simulink model "RI_RL_PI_MRZK_DI"  (R2013b)
settings: Solver=ode45  StartTime=0.0  StopTime=25*L/R  MaxStep=tau/100  RelTol=1e-3
InitFcn:
  | % Modellparaméterek
  | R = 250e-3;
  | L = 10e-3;
  | Psi_0 = 0.5e-3;
  | 
  | i_0 = 0;
  | theta_0 = 0;
  | 
  | % Rendszerparaméterek
  | K = 1/R;
  | tau = L/R;
  | 
  | % PI-hangolás
  | tau_CL = tau/25;
  | xi_CL = 1;
  | 
  | K_PI = (2*xi_CL*tau - tau_CL)/(K*tau_CL);
  | T_I = (2*xi_CL*tau - tau_CL)*tau_CL/tau;
libraries: RI_MK x5, simulink x1
settings Model: Creator=Szalay  LastModifiedBy=Szalay

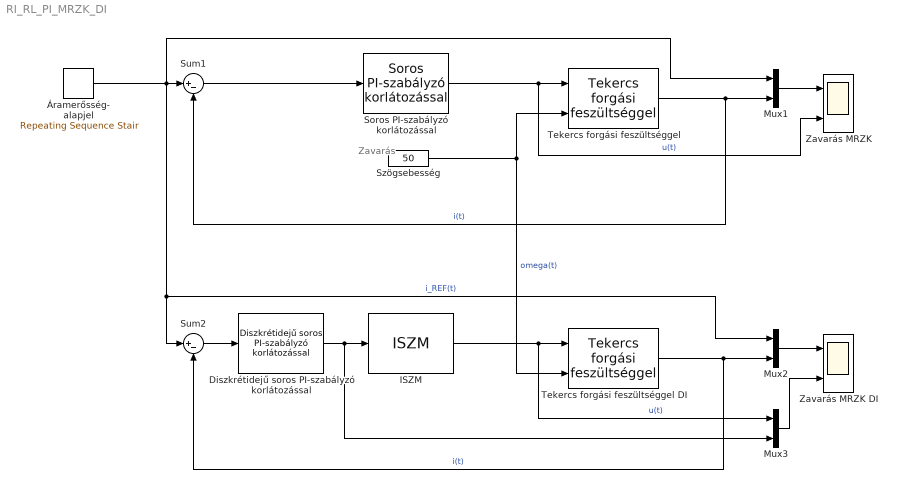
== system RI_RL_PI_MRZK_DI ==
  note: Zavarás
  Diszkrétidejű soros PI-szabályzó korlátozással : RI_MK/Diszkrétidejű soros PI-szabályzó korlátozással  K_PI=K_PI  T_I=T_I  L_U=5  L_L=-5  T_T=T_I  T_S=1/10000/2
  ISZM : RI_MK/ISZM  U_T=5  f_ISZM=10000  T_S=1e-6
  Mux1 : Mux  Inputs=2
  Mux2 : Mux  Inputs=2
  Mux3 : Mux  Inputs=2
  Soros PI-szabályzó korlátozással : RI_MK/Soros PI-szabályzó korlátozással  K_PI=K_PI  T_I=T_I  L_U=5  L_L=-5  T_T=T_I
  Sum1 : Sum  Inputs=|+-
  Sum2 : Sum  Inputs=|+-
  Szögsebesség : Constant  Value=50
  Tekercs forgási feszültséggel : RI_MK/Tekercs forgási feszültséggel  R=R  L=L  Psi_0=Psi_0  i_0=i_0  theta_0=theta_0
  Tekercs forgási feszültséggel DI : RI_MK/Tekercs forgási feszültséggel  R=R  L=L  Psi_0=Psi_0  i_0=i_0  theta_0=theta_0
  Zavarás MRZK : Scope  NumInputPorts=2
      settings: ShowLegends=on  YMin=-5~-5  YMax=5~5
  Zavarás MRZK DI : Scope  NumInputPorts=2
      settings: ShowLegends=on  YMin=-5~-5  YMax=5~5
  Áramerősség- alapjel : simulink/Sources/Repeating Sequence Stair  OutValues=[300, 100, -400, 200, -100]*1e-3  tsamp=L/R*5  OutMin=[]  OutMax=[]  OutDataTypeStr=double  OutputDataTypeScalingMode=double  OutDataType=fixdt(0,8)  ConRadixGroup=Best Precision: Vector-wise  OutScaling=2^-12
  wires:
  Mux1/1 -> Zavarás MRZK/1
  Szögsebesség/1 -> Tekercs forgási feszültséggel DI/2, Tekercs forgási feszültséggel/2  "omega(t)"
  Soros PI-szabályzó korlátozással/1 -> Zavarás MRZK/2, Tekercs forgási feszültséggel/1  "u(t)"
  Tekercs forgási feszültséggel/1 -> Sum1/2, Mux1/2  "i(t)"
  Sum1/1 -> Soros PI-szabályzó korlátozással/1
  Mux2/1 -> Zavarás MRZK DI/1
  ISZM/1 -> Mux3/1, Tekercs forgási feszültséggel DI/1  "u(t)"
  Áramerősség- alapjel/1 -> Mux2/1, Sum2/1, Sum1/1, Mux1/1  "i_REF(t)"
  Tekercs forgási feszültséggel DI/1 -> Mux2/2, Sum2/2  "i(t)"
  Sum2/1 -> Diszkrétidejű soros PI-szabályzó korlátozással/1
  Diszkrétidejű soros PI-szabályzó korlátozással/1 -> Mux3/2, ISZM/1
  Mux3/1 -> Zavarás MRZK DI/2
